simulink model "PID_controller"  (R2019b)
settings: Solver=FixedStepAuto  StartTime=0.0  StopTime=20  FixedStep=0.005  RelTol=1e-3
settings Model: Creator=suvo  LastModifiedBy=suvo

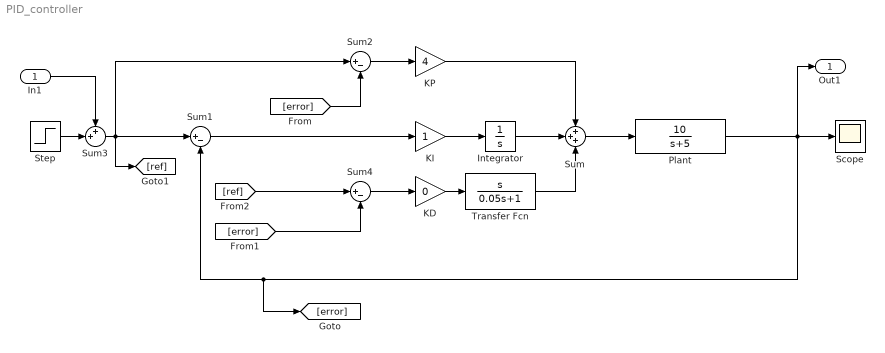
== system PID_controller ==
  In1 : Inport
  Integrator : Integrator
  KD : Gain  Gain=0
  KI : Gain
  KP : Gain  Gain=4
  Plant : TransferFcn  Numerator=10  Denominator=[1 5]
  Scope : Scope
  Step : Step  SampleTime=0
  Sum : Sum  Inputs=+++
  Sum1 : Sum  Inputs=|+-
  Sum2 : Sum  Inputs=|+-
  Sum3 : Sum  Inputs=++|
  Sum4 : Sum  Inputs=|+-
  Transfer Fcn : TransferFcn  Numerator=[1 0]  Denominator=[0.05 1]
  Out1 : Outport
  wires:
  KI/1 -> Integrator/1
  Sum1/1 -> KI/1
  Plant/1 -> Scope/1, Out1/1, [error], Sum1/2
  Sum3/1 -> Sum2/1, Sum1/1, [ref]
  Sum2/1 -> KP/1
  KP/1 -> Sum/1
  Integrator/1 -> Sum/2
  Sum/1 -> Plant/1
  In1/1 -> Sum3/1
  Step/1 -> Sum3/2
  [error] -> Sum2/2
  KD/1 -> Transfer Fcn/1
  Transfer Fcn/1 -> Sum/3
  Sum4/1 -> KD/1
  [error] -> Sum4/2
  [ref] -> Sum4/1
